simulink model "boat_dashboard_trial_3"  (R2021b)
settings: Solver=VariableStepAuto  StartTime=0.0  StopTime=inf  RelTol=1e-3
undefined symbols (not defined in the file): canChannel, DiscIntNeverNeededParam
libraries: canmsglib x16, canlib x13, simulink x3
(part 2 of 2)

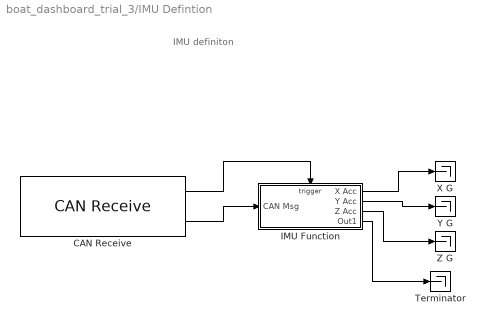
== system boat_dashboard_trial_3/IMU Defintion ==
  note: IMU definiton
  CAN Receive : canlib/CAN Receive  BlockHandle=78.0002  Device=MathWorks Virtual 1 (Channel 1)  DeviceMenu=MathWorks Virtual 1 (Channel 1)  ObjConstructor=canChannel('MathWorks', 'Virtual 1', 1)  EnableStandardIDsFilter=off  StdIDsCombo=Allow all  StandardIDs=1536  EnableExtendedIDsFilter=off  ExtIDsCombo=Allow all  ExtendedIDs=0  SampleTime=0.1  MsgsPerTimestep=all  InternalFilterUpdateStatus=on  BusOutput=off
      settings: SourceProductBaseCode=VN
  IMU Function : Subsystem  TreatAsAtomicUnit=on
  Terminator : Terminator
  X G : Terminator
  Y G : Terminator
  Z G : Terminator
  wires:
  CAN Receive/2 -> IMU Function/1(CAN Msg)
  IMU Function/2(Y Acc) -> Y G/1
  IMU Function/3(Z Acc) -> Z G/1
  CAN Receive/1 -> IMU Function/Trigger
  IMU Function/1(X Acc) -> X G/1
  IMU Function/4(Out1) -> Terminator/1

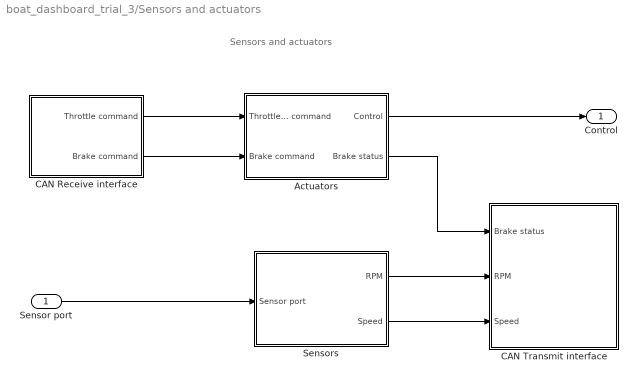
== system boat_dashboard_trial_3/Sensors and actuators ==
  note: Sensors and actuators
  Sensor port : Inport
  Actuators : Subsystem
  CAN Receive interface : Subsystem
  CAN Transmit interface : Subsystem
  Sensors : Subsystem
  Control : Outport  VectorParamsAs1DForOutWhenUnconnected=off
  wires:
  Sensor port/1 -> Sensors/1(Sensor port)
  Sensors/1(RPM) -> CAN Transmit interface/2(RPM)
  Sensors/2(Speed) -> CAN Transmit interface/3(Speed)
  Actuators/1(Control) -> Control/1
  Actuators/2(Brake status) -> CAN Transmit interface/1(Brake status)
  CAN Receive interface/1(Throttle command) -> Actuators/1(Throttle command)
  CAN Receive interface/2(Brake command) -> Actuators/2(Brake command)

== system boat_dashboard_trial_3/Speed controller ==
  note: Speed controller
  CAN Receive : canlib/CAN Receive  BlockHandle=227.0002  Device=MathWorks Virtual 1 (Channel 2)  DeviceMenu=MathWorks Virtual 1 (Channel 2)  ObjConstructor=canChannel('MathWorks', 'Virtual 1', 2)  EnableStandardIDsFilter=off  StdIDsCombo=Allow all  StandardIDs=0  EnableExtendedIDsFilter=off  ExtIDsCombo=Allow all  ExtendedIDs=0  SampleTime=0.01  MsgsPerTimestep=all  InternalFilterUpdateStatus=on  BusOutput=on
      settings: SourceProductBaseCode=VN
  Speed controller ECU logic : Subsystem  TreatAsAtomicUnit=on
  wires:
  CAN Receive/1 -> Speed controller ECU logic/Trigger
  CAN Receive/2 -> Speed controller ECU logic/1(CAN message)

== system boat_dashboard_trial_3/Turn signal ==
  note: Turn signal
  CAN Receive : canlib/CAN Receive  BlockHandle=287.0002  Device=MathWorks Virtual 1 (Channel 2)  DeviceMenu=MathWorks Virtual 1 (Channel 2)  ObjConstructor=canChannel('MathWorks', 'Virtual 1', 2)  EnableStandardIDsFilter=off  StdIDsCombo=Block all  StandardIDs=0  EnableExtendedIDsFilter=off  ExtIDsCombo=Allow all  ExtendedIDs=600  SampleTime=0.01  MsgsPerTimestep=all  InternalFilterUpdateStatus=on  BusOutput=on
      settings: SourceProductBaseCode=VN
  Left turn signal : Terminator
  Right turn signal : Terminator
  Turn signal ECU logic : Subsystem  TreatAsAtomicUnit=on
  wires:
  CAN Receive/1 -> Turn signal ECU logic/Trigger
  CAN Receive/2 -> Turn signal ECU logic/1(CAN message)
  Turn signal ECU logic/1(Left turn signal interface) -> Left turn signal/1
  Turn signal ECU logic/2(Right turn signal interface) -> Right turn signal/1

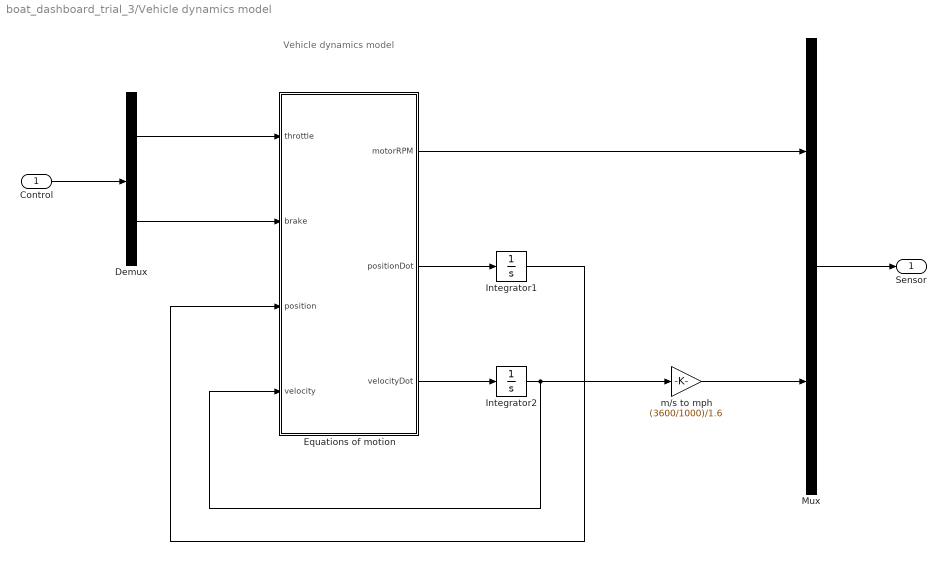
== system boat_dashboard_trial_3/Vehicle dynamics model ==
  note: Vehicle dynamics model
  Control : Inport
  Demux : Demux  Outputs=2
  Equations of motion : MATLAB Function  TreatAsAtomicUnit=on
  Integrator1 : Integrator
  Integrator2 : Integrator
  Mux : Mux  Inputs=2
  m/s to mph : Gain  Gain=(3600/1000)/1.6
  Sensor : Outport  VectorParamsAs1DForOutWhenUnconnected=off
  wires:
  Demux/1 -> Equations of motion/1(throttle)
  Equations of motion/2(positionDot) -> Integrator1/1
  Equations of motion/3(velocityDot) -> Integrator2/1
  Integrator2/1 -> m/s to mph/1, Equations of motion/4(velocity)
  Integrator1/1 -> Equations of motion/3(position)
  Demux/2 -> Equations of motion/2(brake)
  m/s to mph/1 -> Mux/2
  Equations of motion/1(motorRPM) -> Mux/1
  Control/1 -> Demux/1
  Mux/1 -> Sensor/1

== system boat_dashboard_trial_3/Brake light/Brake light ECU logic ==
  note: Brake light ECU logic
  CAN message : Inport
  function : TriggerPort  TriggerType=function-call  VariantControl=Variant
  CAN Unpack : canmsglib/CAN Unpack  CANdbFile=H:\VNT_Project\Cruise_Control\candatabase\canConnectivityForVehicle.dbc  MsgList=BrakeStatusMessage  MsgName=BrakeStatusMessage  MsgIDType=Extended (29-bit identifier)  MsgIdentifier=1280  MsgLength=1  SignalInfo={'BrakeStatus','0','1','LE','unsigned','Standard','0','1','0','0','1'}  IDPort=off  TimestampPort=off  ErrorPort=off  RemotePort=off  LengthPort=off  StatusPort=off  ApplyMinMax=off
      settings: SourceProductBaseCode=ME,XP,VN  DataFormat=CANdb specified signals
  Brake status : Outport  VectorParamsAs1DForOutWhenUnconnected=off
  wires:
  CAN message/1 -> CAN Unpack/1
  CAN Unpack/1 -> Brake status/1

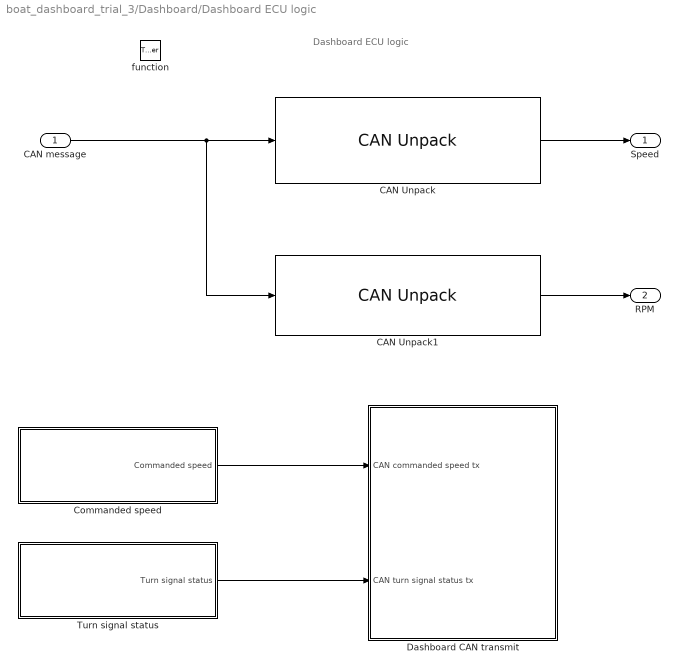
== system boat_dashboard_trial_3/Dashboard/Dashboard ECU logic ==
  note: Dashboard ECU logic
  CAN message : Inport
  function : TriggerPort  TriggerType=function-call  VariantControl=Variant
  CAN Unpack : canmsglib/CAN Unpack  CANdbFile=H:\VNT_Project\Cruise_Control\candatabase\canConnectivityForVehicle.dbc  MsgList=SpeedMessage  MsgName=SpeedMessage  MsgIDType=Extended (29-bit identifier)  MsgIdentifier=256  MsgLength=8  SignalInfo={'Speed','0','64','LE','double','Standard','0','1','0','0','100'}  IDPort=off  TimestampPort=off  ErrorPort=off  RemotePort=off  LengthPort=off  StatusPort=off  ApplyMinMax=off
      settings: SourceProductBaseCode=ME,XP,VN  DataFormat=CANdb specified signals
  CAN Unpack1 : canmsglib/CAN Unpack  CANdbFile=H:\VNT_Project\Cruise_Control\candatabase\canConnectivityForVehicle.dbc  MsgList=RPMMessage  MsgName=RPMMessage  MsgIDType=Extended (29-bit identifier)  MsgIdentifier=2048  MsgLength=8  SignalInfo={'RPM','0','64','LE','double','Standard','0','1','0','0','10000'}  IDPort=off  TimestampPort=off  ErrorPort=off  RemotePort=off  LengthPort=off  StatusPort=off  ApplyMinMax=off
      settings: SourceProductBaseCode=ME,XP,VN  DataFormat=CANdb specified signals
  Commanded speed : Subsystem
  Dashboard CAN transmit : Subsystem
  Turn signal status : Subsystem
  Speed : Outport  VectorParamsAs1DForOutWhenUnconnected=off
  RPM : Outport  Port=2  VectorParamsAs1DForOutWhenUnconnected=off
  wires:
  CAN message/1 -> CAN Unpack1/1, CAN Unpack/1
  Turn signal status/1(Turn signal status) -> Dashboard CAN transmit/2(CAN turn signal status tx)
  Commanded speed/1(Commanded speed) -> Dashboard CAN transmit/1(CAN commanded speed tx)
  CAN Unpack/1 -> Speed/1
  CAN Unpack1/1 -> RPM/1

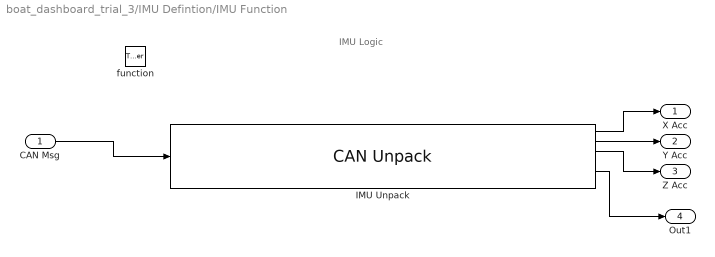
== system boat_dashboard_trial_3/IMU Defintion/IMU Function ==
  note: IMU Logic
  CAN Msg : Inport
  function : TriggerPort  TriggerType=function-call  VariantControl=(inherit)
  IMU Unpack : canmsglib/CAN Unpack  CANdbFile=C:\Users\jerod\OneDrive\Documents\MATLAB\PCAN-GPS_Symbols.dbc  MsgList=BMC_Acceleration  MsgName=BMC_Acceleration  MsgIDType=Standard (11-bit identifier)  MsgIdentifier=1536  MsgLength=8  SignalInfo={'Acceleration_X','0','16','LE','signed','Standard','0','3.91','0','-20000','20000';'Acceleration_Y','16','16','LE','signed','Standard','0','3.91','0','-20000','20000';'Acceleration_Z','32','16','LE','signed','Standard','0','3.91','0','-20000','20000';'Orientation','58','3','LE','unsigned','Standard','0','1','0','0','7';'Temperature','48','8','LE','signed','Standard','0','0.5','24','-40','87.5';'VerticalAxis','56','2','LE','unsigned','Standard','0','1','0','0','3'}  IDPort=off  TimestampPort=off  ErrorPort=off  RemotePort=off  LengthPort=off  StatusPort=off  ApplyMinMax=off
      settings: SourceProductBaseCode=ME,XP,VN  DataFormat=CANdb specified signals
  X Acc : Outport
  Y Acc : Outport  Port=2
  Z Acc : Outport  Port=3
  Out1 : Outport  Port=4
  wires:
  IMU Unpack/3 -> Z Acc/1
  IMU Unpack/1 -> X Acc/1
  IMU Unpack/2 -> Y Acc/1
  CAN Msg/1 -> IMU Unpack/1
  IMU Unpack/5 -> Out1/1

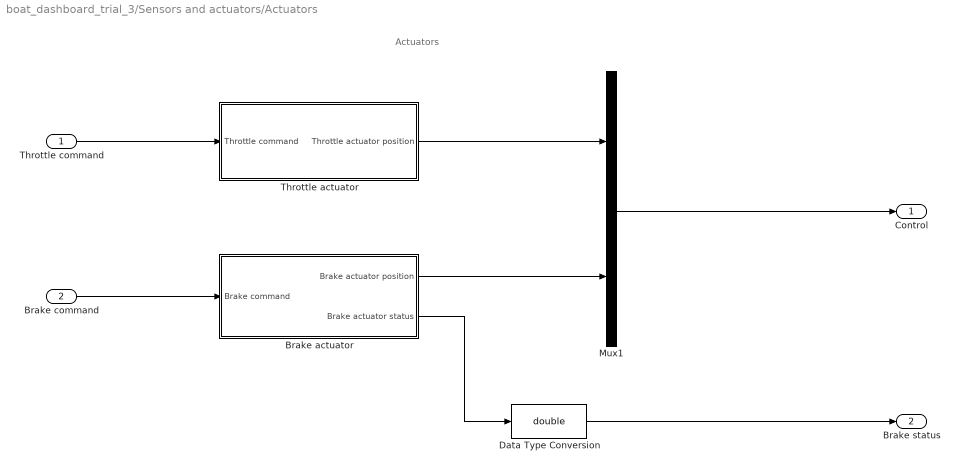
== system boat_dashboard_trial_3/Sensors and actuators/Actuators ==
  note: Actuators
  Throttle command : Inport
  Brake command : Inport  Port=2
  Brake actuator : Subsystem
  Data Type Conversion : DataTypeConversion  OutDataTypeStr=double
  Mux1 : Mux  Inputs=2
  Throttle actuator : Subsystem
  Control : Outport  VectorParamsAs1DForOutWhenUnconnected=off
  Brake status : Outport  Port=2  VectorParamsAs1DForOutWhenUnconnected=off
  wires:
  Brake actuator/1(Brake actuator position) -> Mux1/2
  Throttle actuator/1(Throttle actuator position) -> Mux1/1
  Brake command/1 -> Brake actuator/1(Brake command)
  Throttle command/1 -> Throttle actuator/1(Throttle command)
  Data Type Conversion/1 -> Brake status/1
  Brake actuator/2(Brake actuator status) -> Data Type Conversion/1
  Mux1/1 -> Control/1

== system boat_dashboard_trial_3/Sensors and actuators/CAN Receive interface ==
  note: CAN Receive interface
  CAN Receive : canlib/CAN Receive  BlockHandle=153.0002  Device=MathWorks Virtual 1 (Channel 1)  DeviceMenu=MathWorks Virtual 1 (Channel 1)  ObjConstructor=canChannel('MathWorks', 'Virtual 1', 1)  EnableStandardIDsFilter=off  StdIDsCombo=Allow all  StandardIDs=0  EnableExtendedIDsFilter=off  ExtIDsCombo=Allow all  ExtendedIDs=0  SampleTime=0.01  MsgsPerTimestep=all  InternalFilterUpdateStatus=off  BusOutput=on
      settings: SourceProductBaseCode=VN
  Extract message : Subsystem  TreatAsAtomicUnit=on
  Throttle command : Outport  VectorParamsAs1DForOutWhenUnconnected=off
  Brake command : Outport  Port=2  VectorParamsAs1DForOutWhenUnconnected=off
  wires:
  CAN Receive/1 -> Extract message/Trigger
  CAN Receive/2 -> Extract message/1(In1)
  Extract message/1(Throttle command) -> Throttle command/1
  Extract message/2(Brake actuator position) -> Brake command/1

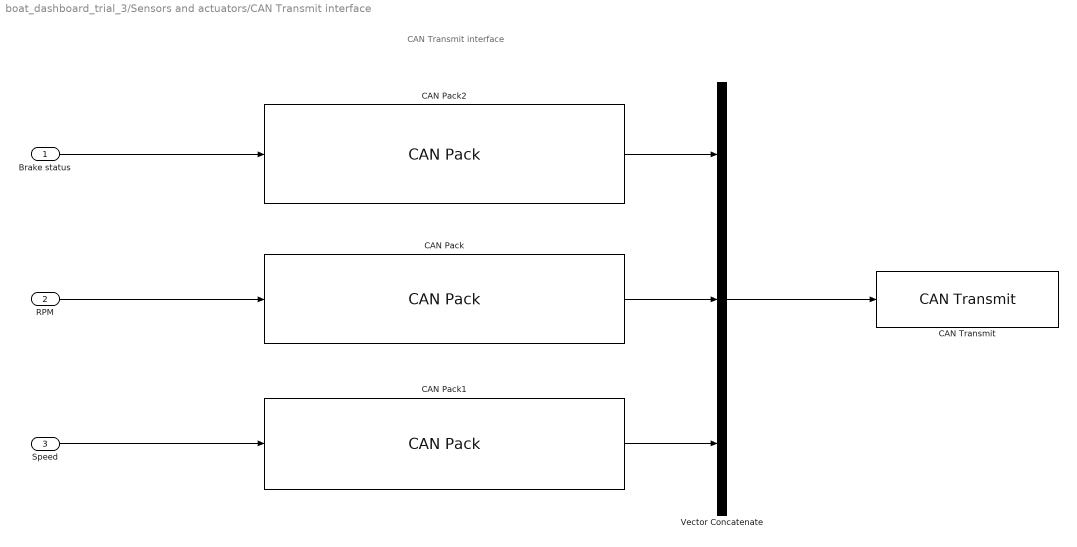
== system boat_dashboard_trial_3/Sensors and actuators/CAN Transmit interface ==
  note: CAN Transmit interface
  Brake status : Inport
  RPM : Inport  Port=2
  Speed : Inport  Port=3
  CAN Pack : canmsglib/CAN Pack  CANdbFile=H:\VNT_Project\Cruise_Control\candatabase\canConnectivityForVehicle.dbc  MsgList=RPMMessage  MsgName=RPMMessage  MsgIDType=Extended (29-bit identifier)  MsgIdentifier=2048  MsgLength=8  Remote=off  ApplyMinMax=off  BusOutput=on  SignalInfo={'RPM','0','64','LE','double','Standard','0','1','0','0','10000'}
      settings: SourceProductBaseCode=ME,XP,VN  DataFormat=CANdb specified signals
  CAN Pack1 : canmsglib/CAN Pack  CANdbFile=H:\VNT_Project\Cruise_Control\candatabase\canConnectivityForVehicle.dbc  MsgList=SpeedMessage  MsgName=SpeedMessage  MsgIDType=Extended (29-bit identifier)  MsgIdentifier=256  MsgLength=8  Remote=off  ApplyMinMax=off  BusOutput=on  SignalInfo={'Speed','0','64','LE','double','Standard','0','1','0','0','100'}
      settings: SourceProductBaseCode=ME,XP,VN  DataFormat=CANdb specified signals
  CAN Pack2 : canmsglib/CAN Pack  CANdbFile=H:\VNT_Project\Cruise_Control\candatabase\canConnectivityForVehicle.dbc  MsgList=BrakeStatusMessage  MsgName=BrakeStatusMessage  MsgIDType=Extended (29-bit identifier)  MsgIdentifier=1280  MsgLength=1  Remote=off  ApplyMinMax=off  BusOutput=on  SignalInfo={'BrakeStatus','0','1','LE','unsigned','Standard','0','1','0','0','1'}
      settings: SourceProductBaseCode=ME,XP,VN  DataFormat=CANdb specified signals
  CAN Transmit : canlib/CAN Transmit  BlockHandle=181.0002  Device=MathWorks Virtual 1 (Channel 1)  DeviceMenu=MathWorks Virtual 1 (Channel 1)  ObjConstructor=canChannel('MathWorks', 'Virtual 1', 1)  EnableEventTransmit=off  EnablePeriodicTransmit=off  MessagePeriod=1.000
      settings: SourceProductBaseCode=VN
  Vector Concatenate : Concatenate  NumInputs=3
  wires:
  Speed/1 -> CAN Pack1/1
  Brake status/1 -> CAN Pack2/1
  CAN Pack1/1 -> Vector Concatenate/3
  Vector Concatenate/1 -> CAN Transmit/1
  CAN Pack/1 -> Vector Concatenate/2
  CAN Pack2/1 -> Vector Concatenate/1
  RPM/1 -> CAN Pack/1

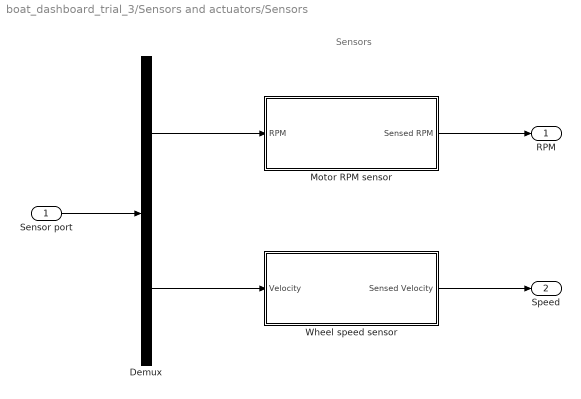
== system boat_dashboard_trial_3/Sensors and actuators/Sensors ==
  note: Sensors
  Sensor port : Inport
  Demux : Demux  Outputs=2
  Motor RPM sensor : Subsystem
  Wheel speed sensor : Subsystem
  RPM : Outport  VectorParamsAs1DForOutWhenUnconnected=off
  Speed : Outport  Port=2  VectorParamsAs1DForOutWhenUnconnected=off
  wires:
  Motor RPM sensor/1(Sensed RPM) -> RPM/1
  Wheel speed sensor/1(Sensed Velocity) -> Speed/1
  Demux/1 -> Motor RPM sensor/1(RPM)
  Demux/2 -> Wheel speed sensor/1(Velocity)
  Sensor port/1 -> Demux/1

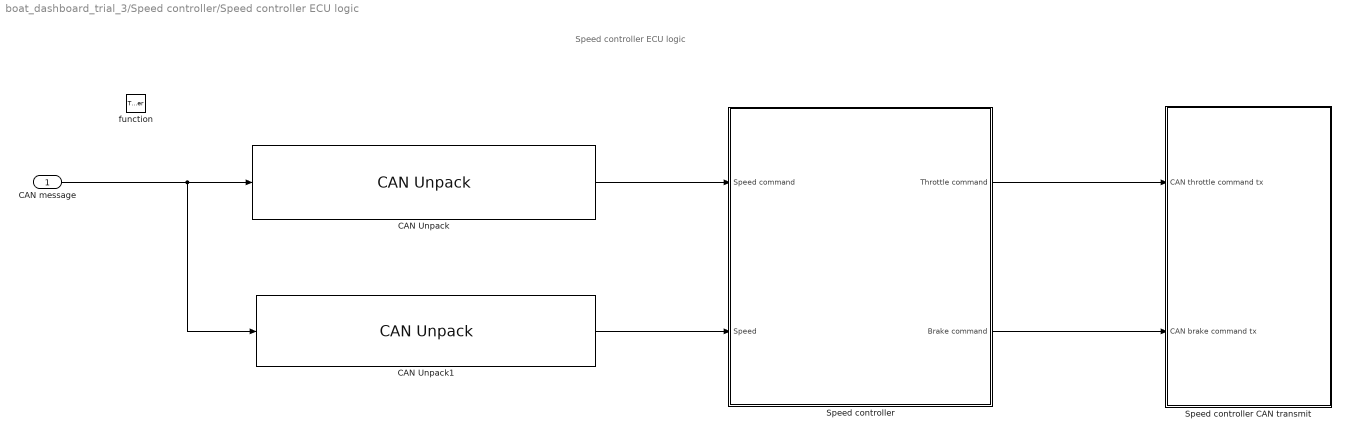
== system boat_dashboard_trial_3/Speed controller/Speed controller ECU logic ==
  note: Speed controller ECU logic
  CAN message : Inport
  function : TriggerPort  TriggerType=function-call  VariantControl=Variant
  CAN Unpack : canmsglib/CAN Unpack  CANdbFile=H:\VNT_Project\Cruise_Control\candatabase\canConnectivityForVehicle.dbc  MsgList=SpeedCommandMessage  MsgName=SpeedCommandMessage  MsgIDType=Extended (29-bit identifier)  MsgIdentifier=1024  MsgLength=8  SignalInfo={'SpeedCommand','0','64','LE','double','Standard','0','1','0','0','100'}  IDPort=off  TimestampPort=off  ErrorPort=off  RemotePort=off  LengthPort=off  StatusPort=off  ApplyMinMax=off
      settings: SourceProductBaseCode=ME,XP,VN  DataFormat=CANdb specified signals
  CAN Unpack1 : canmsglib/CAN Unpack  CANdbFile=H:\VNT_Project\Cruise_Control\candatabase\canConnectivityForVehicle.dbc  MsgList=SpeedMessage  MsgName=SpeedMessage  MsgIDType=Extended (29-bit identifier)  MsgIdentifier=256  MsgLength=8  SignalInfo={'Speed','0','64','LE','double','Standard','0','1','0','0','100'}  IDPort=off  TimestampPort=off  ErrorPort=off  RemotePort=off  LengthPort=off  StatusPort=off  ApplyMinMax=off
      settings: SourceProductBaseCode=ME,XP,VN  DataFormat=CANdb specified signals
  Speed controller : Subsystem
  Speed controller CAN transmit : Subsystem
  wires:
  CAN message/1 -> CAN Unpack1/1, CAN Unpack/1
  Speed controller/1(Throttle command) -> Speed controller CAN transmit/1(CAN throttle command tx)
  Speed controller/2(Brake command) -> Speed controller CAN transmit/2(CAN brake command tx)
  CAN Unpack/1 -> Speed controller/1(Speed command)
  CAN Unpack1/1 -> Speed controller/2(Speed)

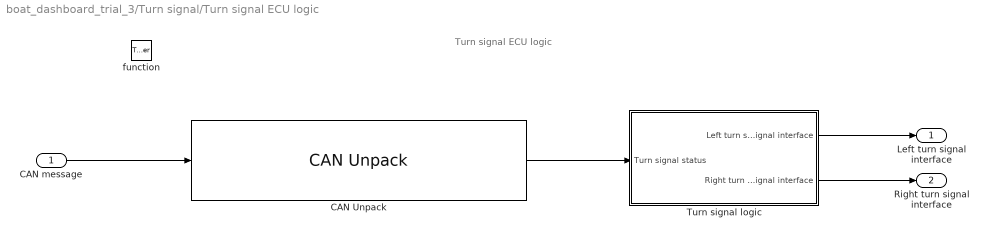
== system boat_dashboard_trial_3/Turn signal/Turn signal ECU logic ==
  note: Turn signal ECU logic
  CAN message : Inport
  function : TriggerPort  TriggerType=function-call  VariantControl=Variant
  CAN Unpack : canmsglib/CAN Unpack  CANdbFile=H:\VNT_Project\Cruise_Control\candatabase\canConnectivityForVehicle.dbc  MsgList=TurnSignalStatusMessage  MsgName=TurnSignalStatusMessage  MsgIDType=Extended (29-bit identifier)  MsgIdentifier=1536  MsgLength=1  SignalInfo={'TurnSignalStatus','0','3','LE','unsigned','Standard','0','1','0','1','3'}  IDPort=off  TimestampPort=off  ErrorPort=off  RemotePort=off  LengthPort=off  StatusPort=off  ApplyMinMax=off
      settings: SourceProductBaseCode=ME,XP,VN  DataFormat=CANdb specified signals
  Turn signal logic : Subsystem
  Left turn signal interface : Outport  VectorParamsAs1DForOutWhenUnconnected=off
  Right turn signal interface : Outport  Port=2  VectorParamsAs1DForOutWhenUnconnected=off
  wires:
  CAN message/1 -> CAN Unpack/1
  CAN Unpack/1 -> Turn signal logic/1(Turn signal status)
  Turn signal logic/1(Left turn signal interface) -> Left turn signal interface/1
  Turn signal logic/2(Right turn signal interface) -> Right turn signal interface/1

== system boat_dashboard_trial_3/Dashboard/Dashboard ECU logic/Commanded speed ==
  note: Commanded speed
  Speed command : Constant  Value=61.59375  OutDataTypeStr=double  SampleTime=Inf
  Zero-Order Hold : ZeroOrderHold  SampleTime=-1
  Commanded speed : Outport  VectorParamsAs1DForOutWhenUnconnected=off
  wires:
  Speed command/1 -> Zero-Order Hold/1
  Zero-Order Hold/1 -> Commanded speed/1

== system boat_dashboard_trial_3/Dashboard/Dashboard ECU logic/Dashboard CAN transmit ==
  note: Dashboard CAN transmit
  CAN commanded speed tx : Inport
  CAN turn signal status tx : Inport  Port=2
  CAN Pack : canmsglib/CAN Pack  CANdbFile=H:\VNT_Project\Cruise_Control\candatabase\canConnectivityForVehicle.dbc  MsgList=TurnSignalStatusMessage  MsgName=TurnSignalStatusMessage  MsgIDType=Extended (29-bit identifier)  MsgIdentifier=1536  MsgLength=1  Remote=off  ApplyMinMax=off  BusOutput=on  SignalInfo={'TurnSignalStatus','0','3','LE','unsigned','Standard','0','1','0','1','3'}
      settings: SourceProductBaseCode=ME,XP,VN  DataFormat=CANdb specified signals
  CAN Pack1 : canmsglib/CAN Pack  CANdbFile=H:\VNT_Project\Cruise_Control\candatabase\canConnectivityForVehicle.dbc  MsgList=SpeedCommandMessage  MsgName=SpeedCommandMessage  MsgIDType=Extended (29-bit identifier)  MsgIdentifier=1024  MsgLength=8  Remote=off  ApplyMinMax=off  BusOutput=on  SignalInfo={'SpeedCommand','0','64','LE','double','Standard','0','1','0','0','100'}
      settings: SourceProductBaseCode=ME,XP,VN  DataFormat=CANdb specified signals
  CAN Transmit : canlib/CAN Transmit  BlockHandle=44.0002  Device=MathWorks Virtual 1 (Channel 1)  DeviceMenu=MathWorks Virtual 1 (Channel 1)  ObjConstructor=canChannel('MathWorks', 'Virtual 1', 1)  EnableEventTransmit=off  EnablePeriodicTransmit=on  MessagePeriod=0.01
      settings: SourceProductBaseCode=VN
  CAN Transmit1 : canlib/CAN Transmit  BlockHandle=45.0002  Device=MathWorks Virtual 1 (Channel 1)  DeviceMenu=MathWorks Virtual 1 (Channel 1)  ObjConstructor=canChannel('MathWorks', 'Virtual 1', 1)  EnableEventTransmit=off  EnablePeriodicTransmit=on  MessagePeriod=0.01
      settings: SourceProductBaseCode=VN
  wires:
  CAN commanded speed tx/1 -> CAN Pack1/1
  CAN Pack/1 -> CAN Transmit/1
  CAN turn signal status tx/1 -> CAN Pack/1
  CAN Pack1/1 -> CAN Transmit1/1

== system boat_dashboard_trial_3/Dashboard/Dashboard ECU logic/Turn signal status ==
  note: Turn signal status
  Turn signal : Constant  Value=2  OutDataTypeStr=double
  Zero-Order Hold : ZeroOrderHold  SampleTime=-1
  Turn signal status : Outport  VectorParamsAs1DForOutWhenUnconnected=off
  wires:
  Turn signal/1 -> Zero-Order Hold/1
  Zero-Order Hold/1 -> Turn signal status/1

== system boat_dashboard_trial_3/Sensors and actuators/Actuators/Brake actuator ==
  note: Brake actuator
  Brake command : Inport
  Brake actuator : TransferFcn  Denominator=[0.1 1]
  Brake status sensor : Subsystem
  Brake actuator position : Outport  VectorParamsAs1DForOutWhenUnconnected=off
  Brake actuator status : Outport  Port=2  VectorParamsAs1DForOutWhenUnconnected=off
  wires:
  Brake status sensor/1(Brake status) -> Brake actuator status/1
  Brake command/1 -> Brake actuator/1
  Brake actuator/1 -> Brake actuator position/1, Brake status sensor/1(Brake actuator position)

== system boat_dashboard_trial_3/Sensors and actuators/Actuators/Throttle actuator ==
  note: Throttle actuator
  Throttle command : Inport
  Throttle actuator : TransferFcn  Denominator=[0.1 1]
  Throttle actuator position : Outport  VectorParamsAs1DForOutWhenUnconnected=off
  wires:
  Throttle command/1 -> Throttle actuator/1
  Throttle actuator/1 -> Throttle actuator position/1

== system boat_dashboard_trial_3/Sensors and actuators/CAN Receive interface/Extract message ==
  note: Extract message
  In1 : Inport
  function : TriggerPort  TriggerType=function-call  VariantControl=Variant
  CAN Unpack : canmsglib/CAN Unpack  CANdbFile=H:\VNT_Project\Cruise_Control\candatabase\canConnectivityForVehicle.dbc  MsgList=ThrottleCommandMessage  MsgName=ThrottleCommandMessage  MsgIDType=Extended (29-bit identifier)  MsgIdentifier=96  MsgLength=8  SignalInfo={'ThrottleCommand','0','64','LE','double','Standard','0','1','0','0','1'}  IDPort=off  TimestampPort=off  ErrorPort=off  RemotePort=off  LengthPort=off  StatusPort=off  ApplyMinMax=off
      settings: SourceProductBaseCode=ME,XP,VN  DataFormat=CANdb specified signals
  CAN Unpack1 : canmsglib/CAN Unpack  CANdbFile=H:\VNT_Project\Cruise_Control\candatabase\canConnectivityForVehicle.dbc  MsgList=BrakeCommandMessage  MsgName=BrakeCommandMessage  MsgIDType=Extended (29-bit identifier)  MsgIdentifier=81  MsgLength=8  SignalInfo={'BrakeCommand','0','64','LE','double','Standard','0','1','0','0','1'}  IDPort=off  TimestampPort=off  ErrorPort=off  RemotePort=off  LengthPort=off  StatusPort=off  ApplyMinMax=off
      settings: SourceProductBaseCode=ME,XP,VN  DataFormat=CANdb specified signals
  Throttle command : Outport  VectorParamsAs1DForOutWhenUnconnected=off
  Brake actuator position : Outport  Port=2  VectorParamsAs1DForOutWhenUnconnected=off
  wires:
  In1/1 -> CAN Unpack1/1, CAN Unpack/1
  CAN Unpack/1 -> Throttle command/1
  CAN Unpack1/1 -> Brake actuator position/1

== system boat_dashboard_trial_3/Sensors and actuators/Sensors/Motor RPM sensor ==
  note: Motor RPM sensor
  RPM : Inport
  Zero-Order Hold : ZeroOrderHold  SampleTime=.01
  Sensed RPM : Outport  VectorParamsAs1DForOutWhenUnconnected=off
  wires:
  Zero-Order Hold/1 -> Sensed RPM/1
  RPM/1 -> Zero-Order Hold/1

== system boat_dashboard_trial_3/Sensors and actuators/Sensors/Wheel speed sensor ==
  note: Wheel speed sensor
  Velocity : Inport
  Zero-Order Hold : ZeroOrderHold  SampleTime=.01
  Sensed Velocity : Outport  VectorParamsAs1DForOutWhenUnconnected=off
  wires:
  Zero-Order Hold/1 -> Sensed Velocity/1
  Velocity/1 -> Zero-Order Hold/1

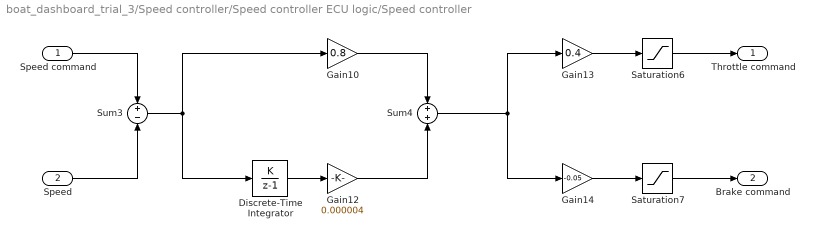
== system boat_dashboard_trial_3/Speed controller/Speed controller ECU logic/Speed controller ==
  Speed command : Inport
  Speed : Inport  Port=2
  Discrete-Time Integrator : DiscreteIntegrator  IntegratorMethod=Accumulation: Forward Euler  SampleTime=-1  ICPrevOutput=DiscIntNeverNeededParam  ICPrevScaledInput=DiscIntNeverNeededParam
  Gain10 : Gain  Gain=0.8
  Gain12 : Gain  Gain=0.000004
  Gain13 : Gain  Gain=0.4
  Gain14 : Gain  Gain=-0.05
  Saturation6 : Saturate  UpperLimit=1  LowerLimit=0
  Saturation7 : Saturate  UpperLimit=1  LowerLimit=0
  Sum3 : Sum  Inputs=+|-
  Sum4 : Sum  Inputs=+|+
  Throttle command : Outport  VectorParamsAs1DForOutWhenUnconnected=off
  Brake command : Outport  Port=2  VectorParamsAs1DForOutWhenUnconnected=off
  wires:
  Saturation7/1 -> Brake command/1
  Saturation6/1 -> Throttle command/1
  Speed command/1 -> Sum3/1
  Speed/1 -> Sum3/2
  Sum3/1 -> Discrete-Time Integrator/1, Gain10/1
  Discrete-Time Integrator/1 -> Gain12/1
  Gain10/1 -> Sum4/1
  Sum4/1 -> Gain14/1, Gain13/1
  Gain14/1 -> Saturation7/1
  Gain13/1 -> Saturation6/1
  Gain12/1 -> Sum4/2

== system boat_dashboard_trial_3/Speed controller/Speed controller ECU logic/Speed controller CAN transmit ==
  CAN throttle command tx : Inport
  CAN brake command tx : Inport  Port=2
  CAN Pack : canmsglib/CAN Pack  CANdbFile=H:\VNT_Project\Cruise_Control\candatabase\canConnectivityForVehicle.dbc  MsgList=ThrottleCommandMessage  MsgName=ThrottleCommandMessage  MsgIDType=Extended (29-bit identifier)  MsgIdentifier=96  MsgLength=8  Remote=off  ApplyMinMax=off  BusOutput=on  SignalInfo={'ThrottleCommand','0','64','LE','double','Standard','0','1','0','0','1'}
      settings: SourceProductBaseCode=ME,XP,VN  DataFormat=CANdb specified signals
  CAN Pack1 : canmsglib/CAN Pack  CANdbFile=H:\VNT_Project\Cruise_Control\candatabase\canConnectivityForVehicle.dbc  MsgList=BrakeCommandMessage  MsgName=BrakeCommandMessage  MsgIDType=Extended (29-bit identifier)  MsgIdentifier=81  MsgLength=8  Remote=off  ApplyMinMax=off  BusOutput=on  SignalInfo={'BrakeCommand','0','64','LE','double','Standard','0','1','0','0','1'}
      settings: SourceProductBaseCode=ME,XP,VN  DataFormat=CANdb specified signals
  CAN Transmit : canlib/CAN Transmit  BlockHandle=267.0002  Device=MathWorks Virtual 1 (Channel 1)  DeviceMenu=MathWorks Virtual 1 (Channel 1)  ObjConstructor=canChannel('MathWorks', 'Virtual 1', 1)  EnableEventTransmit=off  EnablePeriodicTransmit=on  MessagePeriod=0.01
      settings: SourceProductBaseCode=VN
  Vector Concatenate : Concatenate
  wires:
  CAN Pack/1 -> Vector Concatenate/1
  CAN throttle command tx/1 -> CAN Pack/1
  CAN brake command tx/1 -> CAN Pack1/1
  CAN Pack1/1 -> Vector Concatenate/2
  Vector Concatenate/1 -> CAN Transmit/1

== system boat_dashboard_trial_3/Turn signal/Turn signal ECU logic/Turn signal logic ==
  note: Turn signal logic
  Turn signal status : Inport
  Compare To Constant1 : simulink/Logic and Bit Operations/Compare To Constant  relop===  const=1  OutDataTypeStr=boolean
  Compare To Constant2 : simulink/Logic and Bit Operations/Compare To Constant  relop===  const=3  OutDataTypeStr=boolean
  Left turn signal interface : Outport  VectorParamsAs1DForOutWhenUnconnected=off
  Right turn signal interface : Outport  Port=2  VectorParamsAs1DForOutWhenUnconnected=off
  wires:
  Turn signal status/1 -> Compare To Constant2/1, Compare To Constant1/1
  Compare To Constant2/1 -> Right turn signal interface/1
  Compare To Constant1/1 -> Left turn signal interface/1

== system boat_dashboard_trial_3/Sensors and actuators/Actuators/Brake actuator/Brake status sensor ==
  note: Brake status sensor
  Brake actuator position : Inport
  Compare To Constant : simulink/Logic and Bit Operations/Compare To Constant  relop=>  const=0.01  OutDataTypeStr=boolean
  Zero-Order Hold : ZeroOrderHold  SampleTime=0.01
  Brake status : Outport  VectorParamsAs1DForOutWhenUnconnected=off
  wires:
  Zero-Order Hold/1 -> Brake status/1
  Brake actuator position/1 -> Compare To Constant/1
  Compare To Constant/1 -> Zero-Order Hold/1

== matlab function boat_dashboard_trial_3/Vehicle dynamics model/Equations of motion ==
  data: throttle input; brake input; position input; motorRPM output; positionDot output; velocity input; velocityDot output
function [motorRPM, positionDot, velocityDot] = car(throttle, brake, position, velocity) %#ok<INUSL>
% This function defines the equations of motion of the vehicle. The vehicle
% is powered by an electric motor with a gearbox. The gear ratio from the
% motor to the wheels is 6:1.

% Radius of wheel
wheelRadius = 0.3;

% Define the mass properties 
wheelMass = 10;
chassisMass = 1300;
wheelMomentOfInertia = 0.5*wheelMass*wheelRadius*wheelRadius;
mass = (4*wheelMass) + chassisMass + (4 * wheelMomentOfInertia/(wheelRadius^2));

% Compute the motor RPM fromt he wheel speed assuming that the wheels don't
% slip.
motorRPM = (velocity/wheelRadius)*(60/(2*pi))*6;

% Compute the upper bound of the motor torque for the current RPM.
motorTorqueUpperBound = 300*exp(-(0.0001*motorRPM));

% Compute the forces acting on the vehicle.
dragForce = 0.5*1.225*(velocity^2)*2;
totalFrictionForce = 0.4*velocity;
motorForce = throttle*motorTorqueUpperBound*6/wheelRadius;
brakeForce = brake*sign(velocity)*1600/wheelRadius;
force = motorForce - dragForce - totalFrictionForce - brakeForce;

% Equations of motion
positionDot = velocity;
velocityDot = force/mass;
